simulink model "npc_tl_psfb_cdr_final"  (R2024b)
settings: Solver=FixedStepDiscrete  StartTime=0.0  StopTime=8e-3  FixedStep=2e-08  RelTol=1e-3
undefined symbols (not defined in the file): Imag, Real
libraries: spsSeriesRLCBranchLib x12, spsMosfetLib x10, spsDiodeLib x6, spsCurrentMeasurementLib x6, spsVoltageMeasurementLib x6, spsGroundLib x2, spsLinearTransformerLib x1, spsDCVoltageSourceLib x1, sps_lib x1
settings Model: Creator=Open Technical Project  LastModifiedBy=Open Technical Project

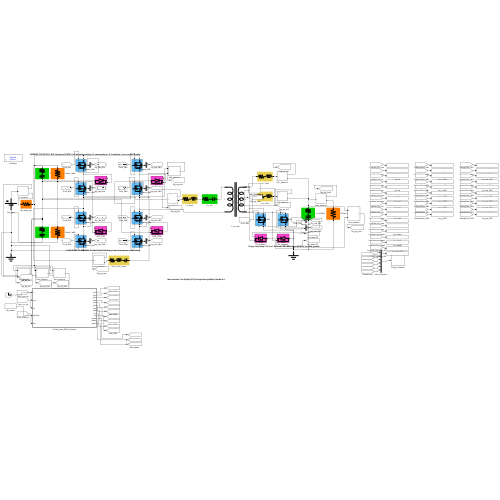
[thumbnail: Simulink's stored preview of the top-level diagram]
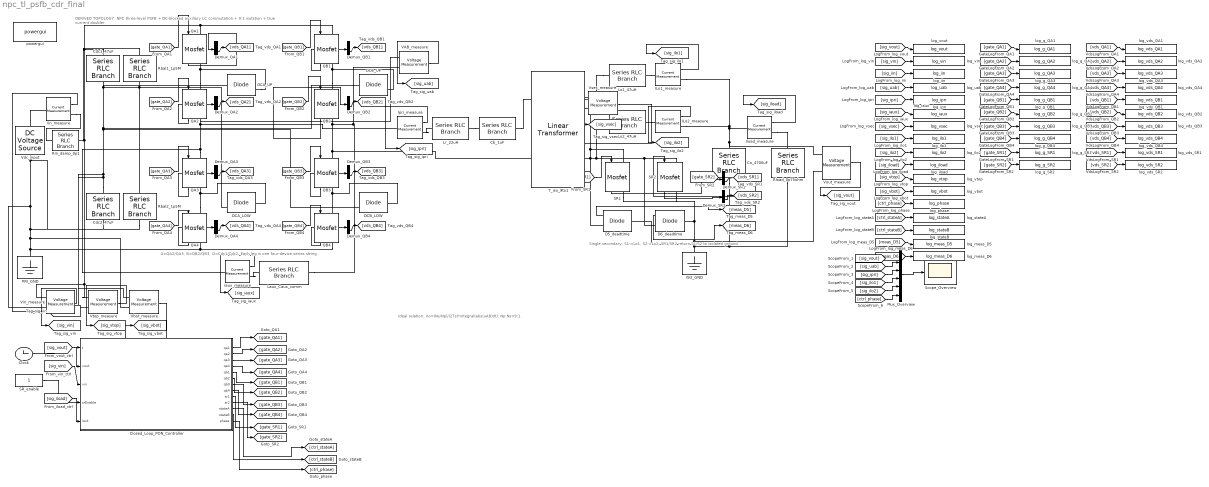
== system npc_tl_psfb_cdr_final ==
  note: DERIVED TOPOLOGY: NPC three-level PSFB + DC-blocked auxiliary LC commutation + 9:1 isolation + true current doubler.
  note: A=QA2/QA3, B=QB2/QB3, O=Cdc1/Cdc2. Each leg is one four-device series string.
  note: Single secondary: S1->Lo1, S2->Lo2; SR1/SR2 return S1/S2 to isolated ground.
  note: Ideal relation: Vo=(Ns/Np)/(2Ts)*integral(abs(uAB)dt); Np:Ns=9:1.
  Cb_1uF : spsSeriesRLCBranchLib/Series RLC Branch  LConnTagsString=__new0  RConnTagsString=__new0  BranchType=RC  Resistance=0.03  Inductance=1e-3  SetiL0=off  InitialCurrent=0  Capacitance=1e-6  Setx0=off  InitialVoltage=0  Measurements=None
  Cdc1_47uF : spsSeriesRLCBranchLib/Series RLC Branch  LConnTagsString=__new0  RConnTagsString=__new0  BranchType=RC  Resistance=0.015  Inductance=1e-3  SetiL0=off  InitialCurrent=0  Capacitance=47e-6  Setx0=off  InitialVoltage=0  Measurements=None
  Cdc2_47uF : spsSeriesRLCBranchLib/Series RLC Branch  LConnTagsString=__new0  RConnTagsString=__new0  BranchType=RC  Resistance=0.015  Inductance=1e-3  SetiL0=off  InitialCurrent=0  Capacitance=47e-6  Setx0=off  InitialVoltage=0  Measurements=None
  Clock : Clock
  Closed_Loop_PON_Controller : MATLAB Function  TreatAsAtomicUnit=on
  Co_4700uF : spsSeriesRLCBranchLib/Series RLC Branch  LConnTagsString=__new0  RConnTagsString=__new0  BranchType=RC  Resistance=0.001  Inductance=1e-3  SetiL0=off  InitialCurrent=0  Capacitance=4700e-6  Setx0=off  InitialVoltage=0  Measurements=None
  D5_deadtime : spsDiodeLib/Diode  Ron=0.003  Lon=0  Vf=0.45  IC=0  UseSnubber=on  Rs=0.1  Cs=180e-12  Measurements=on
  D6_deadtime : spsDiodeLib/Diode  Ron=0.003  Lon=0  Vf=0.45  IC=0  UseSnubber=on  Rs=0.1  Cs=180e-12  Measurements=on
  DCA_LOW : spsDiodeLib/Diode  Ron=0.01  Lon=0  Vf=1.2  IC=0  UseSnubber=on  Rs=0.1  Cs=60e-12  Measurements=on
  DCA_UP : spsDiodeLib/Diode  Ron=0.01  Lon=0  Vf=1.2  IC=0  UseSnubber=on  Rs=0.1  Cs=60e-12  Measurements=on
  DCB_LOW : spsDiodeLib/Diode  Ron=0.01  Lon=0  Vf=1.2  IC=0  UseSnubber=on  Rs=0.1  Cs=60e-12  Measurements=on
  DCB_UP : spsDiodeLib/Diode  Ron=0.01  Lon=0  Vf=1.2  IC=0  UseSnubber=on  Rs=0.1  Cs=60e-12  Measurements=on
  Demux_QA{1..4} (4 alike) : Demux  Outputs=2
  Demux_QB{1..4} (4 alike) : Demux  Outputs=2
  Demux_SR1 : Demux  Outputs=2
  Demux_SR2 : Demux  Outputs=2
  ILo1_measure : spsCurrentMeasurementLib/Current Measurement  PhasorSimulation=off  OutputType=Real-Imag  PSBequivalent=0
  ILo2_measure : spsCurrentMeasurementLib/Current Measurement  PhasorSimulation=off  OutputType=Real-Imag  PSBequivalent=0
  ISO_GND : spsGroundLib/Ground  LConnTagsString=a
  Iaux_measure : spsCurrentMeasurementLib/Current Measurement  PhasorSimulation=off  OutputType=Real-Imag  PSBequivalent=0
  Iin_measure : spsCurrentMeasurementLib/Current Measurement  PhasorSimulation=off  OutputType=Real-Imag  PSBequivalent=0
  Iload_measure : spsCurrentMeasurementLib/Current Measurement  PhasorSimulation=off  OutputType=Real-Imag  PSBequivalent=0
  Ipri_measure : spsCurrentMeasurementLib/Current Measurement  PhasorSimulation=off  OutputType=Real-Imag  PSBequivalent=0
  Laux_Caux_comm : spsSeriesRLCBranchLib/Series RLC Branch  LConnTagsString=__new0  RConnTagsString=__new0  BranchType=RLC  Resistance=0.08  Inductance=200e-6  SetiL0=off  InitialCurrent=0  Capacitance=1e-6  Setx0=off  InitialVoltage=0  Measurements=None
  Lo1_47uH : spsSeriesRLCBranchLib/Series RLC Branch  LConnTagsString=__new0  RConnTagsString=__new0  BranchType=RL  Resistance=0.008  Inductance=47e-6  SetiL0=off  InitialCurrent=0  Capacitance=1e-6  Setx0=off  InitialVoltage=0  Measurements=None
  Lo2_47uH : spsSeriesRLCBranchLib/Series RLC Branch  LConnTagsString=__new0  RConnTagsString=__new0  BranchType=RL  Resistance=0.008  Inductance=47e-6  SetiL0=off  InitialCurrent=0  Capacitance=1e-6  Setx0=off  InitialVoltage=0  Measurements=None
  Lr_22uH : spsSeriesRLCBranchLib/Series RLC Branch  LConnTagsString=__new0  RConnTagsString=__new0  BranchType=RL  Resistance=0.08  Inductance=22e-6  SetiL0=off  InitialCurrent=0  Capacitance=1e-6  Setx0=off  InitialVoltage=0  Measurements=None
  Mux_Overview : Mux  Inputs=6
  PRI_GND : spsGroundLib/Ground  LConnTagsString=a
  QA{1..4} (4 alike) : spsMosfetLib/Mosfet  Ron=0.06  Lon=0  Rd=0.02  Vfd=1.8  IC=0  Rs=0.1  Cs=8e-11  Measurements=on
  QB{1..4} (4 alike) : spsMosfetLib/Mosfet  Ron=0.06  Lon=0  Rd=0.02  Vfd=1.8  IC=0  Rs=0.1  Cs=8e-11  Measurements=on
  Rbal1_1p5M : spsSeriesRLCBranchLib/Series RLC Branch  LConnTagsString=__new0  RConnTagsString=__new0  BranchType=R  Resistance=1.5e6  Inductance=1e-3  SetiL0=off  InitialCurrent=0  Capacitance=1e-6  Setx0=off  InitialVoltage=0  Measurements=None
  Rbal2_1p5M : spsSeriesRLCBranchLib/Series RLC Branch  LConnTagsString=__new0  RConnTagsString=__new0  BranchType=R  Resistance=1.5e6  Inductance=1e-3  SetiL0=off  InitialCurrent=0  Capacitance=1e-6  Setx0=off  InitialVoltage=0  Measurements=None
  Rin_damp_0p1 : spsSeriesRLCBranchLib/Series RLC Branch  LConnTagsString=__new0  RConnTagsString=__new0  BranchType=R  Resistance=0.1  Inductance=1e-3  SetiL0=off  InitialCurrent=0  Capacitance=1e-6  Setx0=off  InitialVoltage=0  Measurements=None
  Rload_0p75ohm : spsSeriesRLCBranchLib/Series RLC Branch  LConnTagsString=__new0  RConnTagsString=__new0  BranchType=R  Resistance=0.75  Inductance=1e-3  SetiL0=off  InitialCurrent=0  Capacitance=1e-6  Setx0=off  InitialVoltage=0  Measurements=None
  SR1 : spsMosfetLib/Mosfet  Ron=0.002  Lon=0  Rd=0.02  Vfd=1.8  IC=0  Rs=0.1  Cs=1.8e-10  Measurements=on
  SR2 : spsMosfetLib/Mosfet  Ron=0.002  Lon=0  Rd=0.02  Vfd=1.8  IC=0  Rs=0.1  Cs=1.8e-10  Measurements=on
  SR_enable : Constant
  Scope_Overview : Scope
  T_iso_9to1 : spsLinearTransformerLib/Linear Transformer  UNITS=SI  NominalPower=[300 150e3]  winding1=[180 0.08 1e-6]  winding2=[20 0.003 50e-9]  ThreeWindings=off  winding3=[3.15e+05 0.7938 0.084225]  RmLm=[2e5 5e-3]  Measurements=None  DataType=on
  VAB_measure : spsVoltageMeasurementLib/Voltage Measurement  PhasorSimulation=off  OutputType=Real-Imag  PSBequivalent=0
  Vbot_measure : spsVoltageMeasurementLib/Voltage Measurement  PhasorSimulation=off  OutputType=Real-Imag  PSBequivalent=0
  Vdc_input : spsDCVoltageSourceLib/DC Voltage Source  Amplitude=740  Measurements=None
  Vin_measure : spsVoltageMeasurementLib/Voltage Measurement  PhasorSimulation=off  OutputType=Real-Imag  PSBequivalent=0
  Vout_measure : spsVoltageMeasurementLib/Voltage Measurement  PhasorSimulation=off  OutputType=Real-Imag  PSBequivalent=0
  Vsec_measure : spsVoltageMeasurementLib/Voltage Measurement  PhasorSimulation=off  OutputType=Real-Imag  PSBequivalent=0
  Vtop_measure : spsVoltageMeasurementLib/Voltage Measurement  PhasorSimulation=off  OutputType=Real-Imag  PSBequivalent=0
  log_g_QA1 : ToWorkspace  VariableName=log_g_QA1  SaveFormat=Structure With Time  SampleTime=-1
  log_g_QA2 : ToWorkspace  VariableName=log_g_QA2  SaveFormat=Structure With Time  SampleTime=-1
  log_g_QA3 : ToWorkspace  VariableName=log_g_QA3  SaveFormat=Structure With Time  SampleTime=-1
  log_g_QA4 : ToWorkspace  VariableName=log_g_QA4  SaveFormat=Structure With Time  SampleTime=-1
  log_g_QB1 : ToWorkspace  VariableName=log_g_QB1  SaveFormat=Structure With Time  SampleTime=-1
  log_g_QB2 : ToWorkspace  VariableName=log_g_QB2  SaveFormat=Structure With Time  SampleTime=-1
  log_g_QB3 : ToWorkspace  VariableName=log_g_QB3  SaveFormat=Structure With Time  SampleTime=-1
  log_g_QB4 : ToWorkspace  VariableName=log_g_QB4  SaveFormat=Structure With Time  SampleTime=-1
  log_g_SR1 : ToWorkspace  VariableName=log_g_SR1  SaveFormat=Structure With Time  SampleTime=-1
  log_g_SR2 : ToWorkspace  VariableName=log_g_SR2  SaveFormat=Structure With Time  SampleTime=-1
  log_iaux : ToWorkspace  VariableName=log_iaux  SaveFormat=Structure With Time  SampleTime=-1
  log_iin : ToWorkspace  VariableName=log_iin  SaveFormat=Structure With Time  SampleTime=-1
  log_ilo1 : ToWorkspace  VariableName=log_ilo1  SaveFormat=Structure With Time  SampleTime=-1
  log_ilo2 : ToWorkspace  VariableName=log_ilo2  SaveFormat=Structure With Time  SampleTime=-1
  log_iload : ToWorkspace  VariableName=log_iload  SaveFormat=Structure With Time  SampleTime=-1
  log_ipri : ToWorkspace  VariableName=log_ipri  SaveFormat=Structure With Time  SampleTime=-1
  log_meas_D5 : ToWorkspace  VariableName=log_meas_D5  SaveFormat=Structure With Time  SampleTime=-1
  log_meas_D6 : ToWorkspace  VariableName=log_meas_D6  SaveFormat=Structure With Time  SampleTime=-1
  log_phase : ToWorkspace  VariableName=log_phase  SaveFormat=Structure With Time  SampleTime=-1
  log_stateA : ToWorkspace  VariableName=log_stateA  SaveFormat=Structure With Time  SampleTime=-1
  log_stateB : ToWorkspace  VariableName=log_stateB  SaveFormat=Structure With Time  SampleTime=-1
  log_uab : ToWorkspace  VariableName=log_uab  SaveFormat=Structure With Time  SampleTime=-1
  log_vbot : ToWorkspace  VariableName=log_vbot  SaveFormat=Structure With Time  SampleTime=-1
  log_vds_QA1 : ToWorkspace  VariableName=log_vds_QA1  SaveFormat=Structure With Time  SampleTime=-1
  log_vds_QA2 : ToWorkspace  VariableName=log_vds_QA2  SaveFormat=Structure With Time  SampleTime=-1
  log_vds_QA3 : ToWorkspace  VariableName=log_vds_QA3  SaveFormat=Structure With Time  SampleTime=-1
  log_vds_QA4 : ToWorkspace  VariableName=log_vds_QA4  SaveFormat=Structure With Time  SampleTime=-1
  log_vds_QB1 : ToWorkspace  VariableName=log_vds_QB1  SaveFormat=Structure With Time  SampleTime=-1
  log_vds_QB2 : ToWorkspace  VariableName=log_vds_QB2  SaveFormat=Structure With Time  SampleTime=-1
  log_vds_QB3 : ToWorkspace  VariableName=log_vds_QB3  SaveFormat=Structure With Time  SampleTime=-1
  log_vds_QB4 : ToWorkspace  VariableName=log_vds_QB4  SaveFormat=Structure With Time  SampleTime=-1
  log_vds_SR1 : ToWorkspace  VariableName=log_vds_SR1  SaveFormat=Structure With Time  SampleTime=-1
  log_vds_SR2 : ToWorkspace  VariableName=log_vds_SR2  SaveFormat=Structure With Time  SampleTime=-1
  log_vin : ToWorkspace  VariableName=log_vin  SaveFormat=Structure With Time  SampleTime=-1
  log_vout : ToWorkspace  VariableName=log_vout  SaveFormat=Structure With Time  SampleTime=-1
  log_vsec : ToWorkspace  VariableName=log_vsec  SaveFormat=Structure With Time  SampleTime=-1
  log_vtop : ToWorkspace  VariableName=log_vtop  SaveFormat=Structure With Time  SampleTime=-1
  powergui : sps_lib/powergui  Priority=1  SimulationMode=Discrete  SampleTime=2e-08  frequency=60  Iterations=50  frequencyindice=0  Pbase=100e6  ErrMax=1e-4  UnitsV=kV  UnitsW=MW  buscounter=0  FunctionMessages=off  echomessages=off  EnableUseOfTLC=off  CurrentSourceSwitches=off  DisableSnubberDevices=off  DisableRonSwitches=off  DisableVfSwitches=off  DisplayEquations=off  AutomaticDiscreteSolvers=off  SolverType=Tustin/Backward Euler (TBE)  Interpol=off  ExternalGateDelay=off  methode=off  Ts=100  x0status=blocks  SPID=on  SwTol=0  HookPort=off  NonlinearTolerance=1e-4  nMaxIteration=100  ContinueOnMaxIteration=off  RestoreLinks=warning  ResistiveCurrentMeasurement=off  Frange=[0:2:500]  Ylog=off  Xlog=on  ShowGrid=off  save=off  variable=ZData  structure=0  ZoomFFT=off  StartTime=0.0  cycles=1  DisplayStyle=1  fundamental=60  FreqAxis=off  MaxFrequency=1000  frequencyindicesteady=1  RmsSteady=1  display=off
  wires:
  Clock/1 -> Closed_Loop_PON_Controller/1(t)
  Vin_measure/1 -> [sig_vin]
  Iin_measure/1 -> [sig_iin]
  Vout_measure/1 -> [sig_vout]
  Vtop_measure/1 -> [sig_vtop]
  Vbot_measure/1 -> [sig_vbot]
  VAB_measure/1 -> [sig_uab]
  Vsec_measure/1 -> [sig_vsec]
  Ipri_measure/1 -> [sig_ipri]
  Iaux_measure/1 -> [sig_iaux]
  ILo1_measure/1 -> [sig_ilo1]
  ILo2_measure/1 -> [sig_ilo2]
  Iload_measure/1 -> [sig_iload]
  [sig_vout] -> Closed_Loop_PON_Controller/2(vout)
  [sig_vin] -> Closed_Loop_PON_Controller/3(vin)
  SR_enable/1 -> Closed_Loop_PON_Controller/4(srEnable)
  [sig_iload] -> Closed_Loop_PON_Controller/5(iout)
  Closed_Loop_PON_Controller/1(qa1) -> [gate_QA1]
  Closed_Loop_PON_Controller/2(qa2) -> [gate_QA2]
  Closed_Loop_PON_Controller/3(qa3) -> [gate_QA3]
  Closed_Loop_PON_Controller/4(qa4) -> [gate_QA4]
  Closed_Loop_PON_Controller/5(qb1) -> [gate_QB1]
  Closed_Loop_PON_Controller/6(qb2) -> [gate_QB2]
  Closed_Loop_PON_Controller/7(qb3) -> [gate_QB3]
  Closed_Loop_PON_Controller/8(qb4) -> [gate_QB4]
  Closed_Loop_PON_Controller/9(sr1) -> [gate_SR1]
  Closed_Loop_PON_Controller/10(sr2) -> [gate_SR2]
  [gate_QA1] -> QA1/1
  [gate_QA2] -> QA2/1
  [gate_QA3] -> QA3/1
  [gate_QA4] -> QA4/1
  [gate_QB1] -> QB1/1
  [gate_QB2] -> QB2/1
  [gate_QB3] -> QB3/1
  [gate_QB4] -> QB4/1
  [gate_SR1] -> SR1/1
  [gate_SR2] -> SR2/1
  D5_deadtime/1 -> [meas_D5]
  D6_deadtime/1 -> [meas_D6]
  Closed_Loop_PON_Controller/11(stateA) -> [ctrl_stateA]
  Closed_Loop_PON_Controller/12(stateB) -> [ctrl_stateB]
  Closed_Loop_PON_Controller/13(phase) -> [ctrl_phase]
  QA1/1 -> Demux_QA1/1
  Demux_QA1/2 -> [vds_QA1]
  QA2/1 -> Demux_QA2/1
  Demux_QA2/2 -> [vds_QA2]
  QA3/1 -> Demux_QA3/1
  Demux_QA3/2 -> [vds_QA3]
  QA4/1 -> Demux_QA4/1
  Demux_QA4/2 -> [vds_QA4]
  QB1/1 -> Demux_QB1/1
  Demux_QB1/2 -> [vds_QB1]
  QB2/1 -> Demux_QB2/1
  Demux_QB2/2 -> [vds_QB2]
  QB3/1 -> Demux_QB3/1
  Demux_QB3/2 -> [vds_QB3]
  QB4/1 -> Demux_QB4/1
  Demux_QB4/2 -> [vds_QB4]
  SR1/1 -> Demux_SR1/1
  Demux_SR1/2 -> [vds_SR1]
  SR2/1 -> Demux_SR2/1
  Demux_SR2/2 -> [vds_SR2]
  [sig_vout] -> log_vout/1
  [sig_vin] -> log_vin/1
  [sig_iin] -> log_iin/1
  [sig_uab] -> log_uab/1
  [sig_ipri] -> log_ipri/1
  [sig_iaux] -> log_iaux/1
  [sig_vsec] -> log_vsec/1
  [sig_ilo1] -> log_ilo1/1
  [sig_ilo2] -> log_ilo2/1
  [sig_iload] -> log_iload/1
  [sig_vtop] -> log_vtop/1
  [sig_vbot] -> log_vbot/1
  [ctrl_phase] -> log_phase/1
  [ctrl_stateA] -> log_stateA/1
  [ctrl_stateB] -> log_stateB/1
  [meas_D5] -> log_meas_D5/1
  [meas_D6] -> log_meas_D6/1
  [gate_QA1] -> log_g_QA1/1
  [vds_QA1] -> log_vds_QA1/1
  [gate_QA2] -> log_g_QA2/1
  [vds_QA2] -> log_vds_QA2/1
  [gate_QA3] -> log_g_QA3/1
  [vds_QA3] -> log_vds_QA3/1
  [gate_QA4] -> log_g_QA4/1
  [vds_QA4] -> log_vds_QA4/1
  [gate_QB1] -> log_g_QB1/1
  [vds_QB1] -> log_vds_QB1/1
  [gate_QB2] -> log_g_QB2/1
  [vds_QB2] -> log_vds_QB2/1
  [gate_QB3] -> log_g_QB3/1
  [vds_QB3] -> log_vds_QB3/1
  [gate_QB4] -> log_g_QB4/1
  [vds_QB4] -> log_vds_QB4/1
  [gate_SR1] -> log_g_SR1/1
  [vds_SR1] -> log_vds_SR1/1
  [gate_SR2] -> log_g_SR2/1
  [vds_SR2] -> log_vds_SR2/1
  [sig_vout] -> Mux_Overview/1
  [sig_uab] -> Mux_Overview/2
  [sig_ipri] -> Mux_Overview/3
  [sig_ilo1] -> Mux_Overview/4
  [sig_ilo2] -> Mux_Overview/5
  [ctrl_phase] -> Mux_Overview/6
  Mux_Overview/1 -> Scope_Overview/1
  connections:
  Vdc_input/RConn1 -- Iin_measure/LConn1
  Iin_measure/RConn1 -- Rin_damp_0p1/LConn1
  Cdc1_47uF/LConn1 -- QB1/LConn1 -- QA1/LConn1 -- Vin_measure/LConn1 -- Vtop_measure/LConn1 -- Rin_damp_0p1/RConn1 -- Rbal1_1p5M/LConn1
  Cdc2_47uF/LConn1 -- DCA_LOW/RConn1 -- Rbal1_1p5M/RConn1 -- Rbal2_1p5M/LConn1 -- Cdc1_47uF/RConn1 -- DCA_UP/LConn1 -- DCB_UP/LConn1 -- DCB_LOW/RConn1 -- Vbot_measure/LConn1 -- Vtop_measure/LConn2
  Cdc2_47uF/RConn1 -- Vbot_measure/LConn2 -- QB4/RConn1 -- QA4/RConn1 -- PRI_GND/LConn1 -- Vdc_input/LConn1 -- Rbal2_1p5M/RConn1 -- Vin_measure/LConn2
  QA2/LConn1 -- QA1/RConn1 -- DCA_UP/RConn1
  QA3/LConn1 -- QA2/RConn1 -- Ipri_measure/LConn1 -- VAB_measure/LConn1 -- Iaux_measure/LConn1
  QA4/LConn1 -- QA3/RConn1 -- DCA_LOW/LConn1
  QB2/LConn1 -- QB1/RConn1 -- DCB_UP/RConn1
  QB3/LConn1 -- Laux_Caux_comm/RConn1 -- VAB_measure/LConn2 -- QB2/RConn1 -- T_iso_9to1/LConn2
  QB4/LConn1 -- QB3/RConn1 -- DCB_LOW/LConn1
  Ipri_measure/RConn1 -- Lr_22uH/LConn1
  Lr_22uH/RConn1 -- Cb_1uF/LConn1
  Cb_1uF/RConn1 -- T_iso_9to1/LConn1
  Iaux_measure/RConn1 -- Laux_Caux_comm/LConn1
  Lo1_47uH/LConn1 -- D5_deadtime/RConn1 -- SR1/LConn1 -- T_iso_9to1/RConn1 -- Vsec_measure/LConn1
  Lo2_47uH/LConn1 -- T_iso_9to1/RConn2 -- Vsec_measure/LConn2 -- D6_deadtime/RConn1 -- SR2/LConn1
  Lo1_47uH/RConn1 -- ILo1_measure/LConn1
  Lo2_47uH/RConn1 -- ILo2_measure/LConn1
  ILo1_measure/RConn1 -- ILo2_measure/RConn1 -- Iload_measure/LConn1 -- Co_4700uF/LConn1 -- Vout_measure/LConn1
  SR1/RConn1 -- ISO_GND/LConn1 -- Rload_0p75ohm/RConn1 -- Co_4700uF/RConn1 -- SR2/RConn1 -- D5_deadtime/LConn1 -- Vout_measure/LConn2 -- D6_deadtime/LConn1
  Iload_measure/RConn1 -- Rload_0p75ohm/LConn1

== matlab function npc_tl_psfb_cdr_final/Closed_Loop_PON_Controller ==
  data: t input; qa1 output; vout input; vin input; srEnable input; iout input; qa2 output; qa3 output; qa4 output; qb1 output; qb2 output; qb3 output; qb4 output; sr1 output; sr2 output; stateA output; stateB output; phase output
function [qa1,qa2,qa3,qa4,qb1,qb2,qb3,qb4,sr1,sr2,stateA,stateB,phase] = ctrl(t,vout,vin,srEnable,iout)
                                                                                                      %#codegen                                                                                              
                                                                                                      persistent integ phaseHold lastCycle burstOn ioutFilt lightMode voutPrev                               
                                                                                                      fs = 150e3;                                                                                            
                                                                                                      T = 1/fs;                                                                                              
                                                                                                      zeroDwell = 0.025;                                                                                     
                                                                                                      deadNorm = 220e-9/T;                                                                                   
                                                                                                      Nps = 9;                                                                                               
                                                                                                      if isempty(lastCycle)                                                                                  
                                                                                                          integ = 0; phaseHold = 0.05; lastCycle = -1; burstOn = true;                                       
                                                                                                          ioutFilt = 0; lightMode = false; voutPrev = 0;                                                     
                                                                                                      end                                                                                                    
                                                                                                      cycle = floor(t/T);                                                                                    
                                                                                                      if cycle ~= lastCycle                                                                                  
                                                                                                          ramp = min(t/1e-3,1);                                                                              
                                                                                                          if t < 1e-3 && vout > 14, ramp = 1; end                                                            
                                                                                                          vref = 15*ramp;                                                                                    
                                                                                                          err = vref-vout;                                                                                   
                                                                                                          ioutFilt = 0.98*ioutFilt+0.02*max(iout,0);                                                         
                                                                                                          dvCycle = vout-voutPrev;                                                                           
                                                                                                          if t > 5e-3                                                                                        
                                                                                                              if ioutFilt < 5.2 && abs(dvCycle) < 5e-3 && vout > 14.8                                        
                                                                                                                  lightMode = true;                                                                          
                                                                                                              end                                                                                            
                                                                                                              if ioutFilt > 6.0, lightMode = false; end                                                      
                                                                                                          end                                                                                                
                                                                                                          if ~lightMode || burstOn                                                                           
                                                                                                              integ = integ+err*T;                                                                           
                                                                                                          end                                                                                                
                                                                                                          integ = min(max(integ,-0.012),0.012);                                                              
                                                                                                          gainScale = min(1,350/max(vin,350));                                                               
                                                                                                          phaseFF = Nps*vref/max(vin,50)+(10/max(vin,50)+0.004)*ramp;                                        
                                                                                                          cmd = phaseFF+0.0025*gainScale*err+8*gainScale*integ;                                              
                                                                                                          phaseHold = min(max(cmd,0.03),0.45);                                                               
                                                                                                          if lightMode                                                                                       
                                                                                                              if vout >= 15.008, burstOn = false; end                                                        
                                                                                                              if vout <= 14.992, burstOn = true; end                                                         
                                                                                                          else                                                                                               
                                                                                                              burstOn = true;                                                                                
                                                                                                          end                                                                                                
                                                                                                          voutPrev = vout;                                                                                   
                                                                                                          lastCycle = cycle;                                                                                 
                                                                                                      end                                                                                                    
                                                                                                      phase = phaseHold;                                                                                     
                                                                                                      if ~burstOn                                                                                            
                                                                                                          qa1=0; qa2=1; qa3=1; qa4=0;                                                                        
                                                                                                          qb1=0; qb2=1; qb3=1; qb4=0;                                                                        
                                                                                                          sr1=0; sr2=0; stateA=0; stateB=0;                                                                  
                                                                                                          return;                                                                                            
                                                                                                      end                                                                                                    
                                                                                                      pA = t/T-floor(t/T);                                                                                   
                                                                                                      pB = pA-phaseHold;                                                                                     
                                                                                                      if pB < 0, pB = pB+1; end                                                                              
                                                                                                      [qa1,qa2,qa3,qa4,stateA] = leg_gate(pA,zeroDwell,deadNorm);                                            
                                                                                                      [qb1,qb2,qb3,qb4,stateB] = leg_gate(pB,zeroDwell,deadNorm);                                            
                                                                                                      delta = stateA-stateB;                                                                                 
                                                                                                      if srEnable < 0.5                                                                                      
                                                                                                          sr1=0; sr2=0;                                                                                      
                                                                                                      elseif delta > 0.5                                                                                     
                                                                                                          sr1=0; sr2=1;                                                                                      
                                                                                                      elseif delta < -0.5                                                                                    
                                                                                                          sr1=1; sr2=0;                                                                                      
                                                                                                      else                                                                                                   
                                                                                                          sr1=1; sr2=1;                                                                                      
                                                                                                      end                                                                                                    
                                                                                                      end                                                                                                    
                                                                                                                                                                                                             
                                                                                                      function [q1,q2,q3,q4,state] = leg_gate(p,z,td)                                                        
                                                                                                      q1=0; q2=0; q3=0; q4=0; state=0;                                                                       
                                                                                                      if p < z                                                                                               
                                                                                                          q2=1; q3=1;                                                                                        
                                                                                                      elseif p < z+td                                                                                        
                                                                                                          q2=1;                                                                                              
                                                                                                      elseif p < 0.5-z                                                                                       
                                                                                                          q1=1; q2=1; state=1;                                                                               
                                                                                                      elseif p < 0.5-z+td                                                                                    
                                                                                                          q2=1;                                                                                              
                                                                                                      elseif p < 0.5+z                                                                                       
                                                                                                          q2=1; q3=1;                                                                                        
                                                                                                      elseif p < 0.5+z+td                                                                                    
                                                                                                          q3=1;                                                                                              
                                                                                                      elseif p < 1-z                                                                                         
                                                                                                          q3=1; q4=1; state=-1;                                                                              
                                                                                                      elseif p < 1-z+td                                                                                      
                                                                                                          q3=1;                                                                                              
                                                                                                      else                                                                                                   
                                                                                                          q2=1; q3=1;                                                                                        
                                                                                                      end                                                                                                    
                                                                                                      end
